simulink model "Average"  (R2021a)
settings: Solver=FixedStepDiscrete  StartTime=0.0  StopTime=10.0  RelTol=1e-3
settings Model: Creator=Moamen_Hamed  LastModifiedBy=Mahmoud Shams El-Din
settings OptimizationCC: BlockReduction=off  DefaultParameterBehavior=Inlined  EnhancedBackFolding=on  PassReuseOutputArgsAs=Individual arguments  OptimizeBlockOrder=speed  DifferentSizesBufferReuse=on  OptimizationCustomize=off  EfficientTunableParamExpr=on
settings DebuggingCC: ParameterTunabilityLossMsg=error
settings SFSimCC: MATLABDynamicMemAlloc=off
settings RTWCC: SystemTargetFile=ert.tlc  GenCodeOnly=on  TemplateMakefile=ert_default_tmf  GenerateReport=on  IncludeHyperlinkInReport=on  LaunchReport=on  GenerateTraceInfo=on
settings CodeAppCC: ForceParamTrailComments=on  IgnoreCustomStorageClasses=off  OperatorAnnotations=on  SimulinkDataObjDesc=on  SFDataObjDesc=on  InsertBlockDesc=on
settings ERTTargetCC: TargetLangStandard=C99 (ISO)  GenerateSampleERTMain=on  CodeInterfacePackaging=Reusable function  SupportComplex=off  InlinedParameterPlacement=NonHierarchical  ERTCustomFileTemplate=example_file_process.tlc

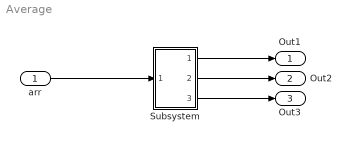
== system Average ==
  arr : Inport  PortDimensions=10
  Subsystem : Subsystem  TreatAsAtomicUnit=on
  Out1 : Outport  SignalName=Avr_Out
  Out2 : Outport  Port=2  SignalName=Max_Out
  Out3 : Outport  Port=3  SignalName=Min_Out
  wires:
  arr/1 -> Subsystem/1(In1)
  Subsystem/1(Out1) -> Out1/1
  Subsystem/2(Out2) -> Out2/1
  Subsystem/3(Out3) -> Out3/1

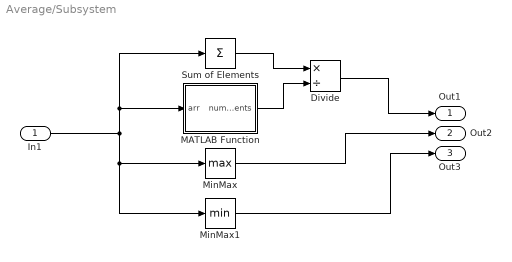
== system Average/Subsystem ==
  In1 : Inport
  Divide : Product  Inputs=*/
  MATLAB Function : MATLAB Function  TreatAsAtomicUnit=on
  MinMax : MinMax  Function=max
  MinMax1 : MinMax
  Sum of Elements : Sum  Inputs=+
  Out1 : Outport
  Out2 : Outport  Port=2
  Out3 : Outport  Port=3
  wires:
  In1/1 -> MinMax1/1, MinMax/1, MATLAB Function/1(arr), Sum of Elements/1
  Divide/1 -> Out1/1
  MATLAB Function/1(numElements) -> Divide/2
  Sum of Elements/1 -> Divide/1
  MinMax1/1 -> Out3/1
  MinMax/1 -> Out2/1

== matlab function Average/Subsystem/MATLAB Function ==
  data: arr input; numElements output
function numElements = array_length(arr)
    numElements = numel(arr);
end
